simulink model "me132LabPartE"  (R2021a)
settings: Solver=VariableStepAuto  StartTime=0.0  StopTime=10.0  MaxStep=0.02  RelTol=1e-3
undefined symbols (not defined in the file or in its folder): c3
settings Model: Creator=kaiyu  LastModifiedBy=kaiyu

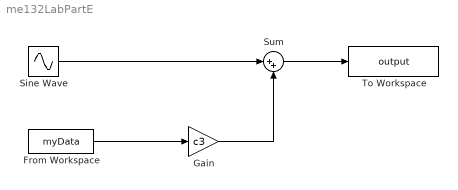
== system me132LabPartE ==
  From Workspace : FromWorkspace  VariableName=myData
  Gain : Gain  Gain=c3
  Sine Wave : Sin  Amplitude=0.2  Frequency=10  SampleTime=0
  Sum : Sum  Inputs=|++
  To Workspace : ToWorkspace  VariableName=output  SaveFormat=Structure With Time  SampleTime=-1
  wires:
  From Workspace/1 -> Gain/1
  Gain/1 -> Sum/2
  Sine Wave/1 -> Sum/1
  Sum/1 -> To Workspace/1
